simulink subsystem "ParametricTwoFingerGripperSubsystem"  (R2024a)
settings: Solver=VariableStepAuto  StartTime=0.0  StopTime=10.0  RelTol=1e-3
PostLoadFcn:
  | ParametricGripperPayloadsParameters
undefined symbols (not defined in the file): F1, F2
libraries: GripperLib x1
settings Model: Creator=abirdas  LastModifiedBy=abirdas
settings RTWCC: GPUComputeCapability=3.5

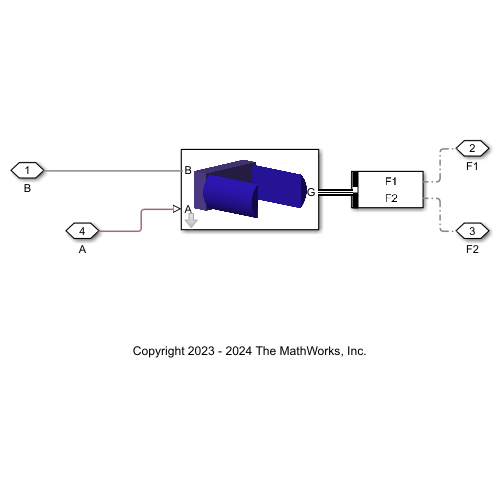
[thumbnail: Simulink's stored preview of the top-level diagram]
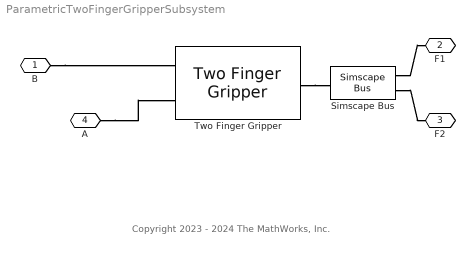
== system ParametricTwoFingerGripperSubsystem ==
  note: Copyright 2023 - 2024 The MathWorks, Inc.
  Simscape Bus : SimscapeBus  HierarchyStrings=F1;F2
  Two Finger Gripper : GripperLib/Two Finger Gripper  lFinger=ParametricRobot.Gripper.FingerLength  wFinger=ParametricRobot.Gripper.FingerWidth  sFingerMax=ParametricRobot.Gripper.FingerMaxOpening  kFingerJoint=ParametricRobot.Gripper.JointStiffness  colorFinger=ParametricRobot.Gripper.FingerColor  ptcldDensity=fingerPointCloudDensity
  B : PMIOPort  Side=Left
  F1 : PMIOPort  Port=2  Side=Right
  F2 : PMIOPort  Port=3  Side=Right
  A : PMIOPort  Port=4  Side=Left
  connections:
  Simscape Bus/LConn1 -- F1/RConn1
  Two Finger Gripper/RConn1 -- Simscape Bus/RConn1
  Simscape Bus/LConn2 -- F2/RConn1
  A/RConn1 -- Two Finger Gripper/LConn2
  B/RConn1 -- Two Finger Gripper/LConn1
